simulink model "Pump_comparison"  (R2018b)
settings: Solver=VariableStepAuto  StartTime=0.0  StopTime=200  MaxStep=5  RelTol=1e-3  EnableMultiTasking=on
undefined symbols (not defined in the file): ID, MassFlow, path_carnot, Pressure, Temperature, Water
libraries: carnot x8, simulink x1
settings Model: Creator=drhf  LastModifiedBy=drhf
settings DataIOCC: LimitDataPoints=on  SaveFormat=Array  SignalLoggingSaveFormat=ModelDataLogs
settings OptimizationCC: ExpressionDepthLimit=2147483647  LifeSpan=inf
settings DebuggingCC: UnderspecifiedInitializationDetection=Classic  MergeDetectMultiDrivingBlocksExec=none  SolverPrmCheckMsg=warning  StateNameClashWarn=warning  SFUnexpectedBacktrackingDiag=warning  SFNoUnconditionalDefaultTransitionDiag=warning  SFExecutionAtInitializationDiag=none
settings HardwareCC: ProdBitPerPointer=32  ProdBitPerSizeT=32  ProdBitPerPtrDiffT=32  ProdLargestAtomicFloat=None  ProdIntDivRoundTo=Undefined  ProdEndianess=Unspecified  ProdWordSize=32  ProdHWDeviceType=32-bit Generic
settings ModelReferenceCC: PropagateSignalLabelsOutOfModel=off
settings SFSimCC: SimUseLocalCustomCode=off
settings RTWCC: RTWUseLocalCustomCode=off
settings CodeAppCC: StateflowObjectComments=on
settings GRTTargetCC: TargetLangStandard=C89/C90 (ANSI)  GeneratePreprocessorConditionals=Disable all  CombineOutputUpdateFcns=off  GRTInterface=on
settings ConfigComp: CovMetricSettings=dw  CovHtmlReporting=on  CovSaveCumulativeToWorkspaceVar=on  CovSaveSingleToWorkspaceVar=on  CovExternalEMLEnable=off

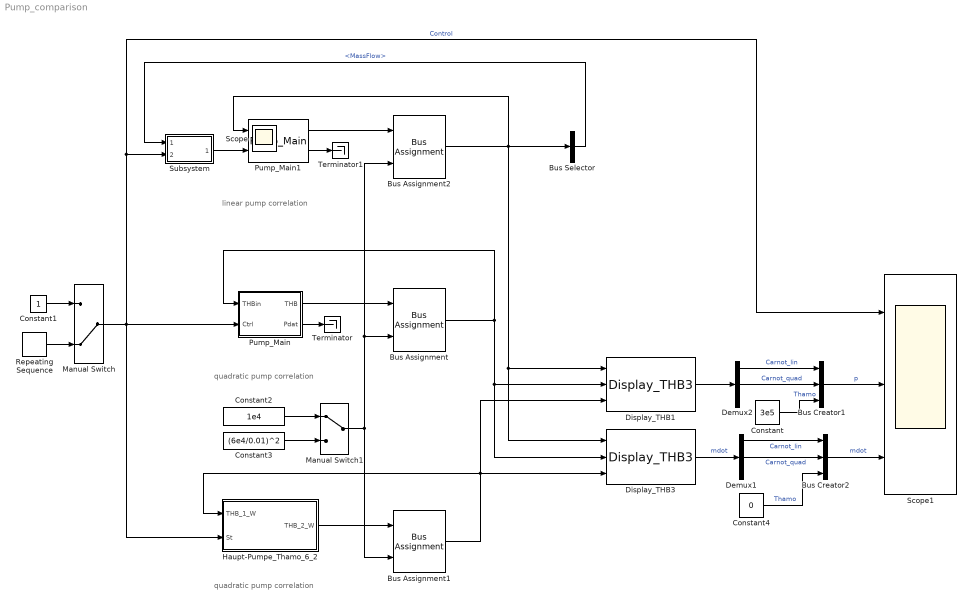
== system Pump_comparison ==
  note: quadratic pump correlation
  note: quadratic pump correlation
  note: linear pump correlation
  Bus Assignment : BusAssignment  AssignedSignals=DPQuadratic
  Bus Assignment1 : BusAssignment  AssignedSignals=DPQuadratic
  Bus Assignment2 : BusAssignment  AssignedSignals=DPQuadratic
  Bus Creator1 : BusCreator  Inputs=3
  Bus Creator2 : BusCreator  Inputs=3
  Bus Selector : BusSelector  OutputSignals=MassFlow
  Constant : Constant  Value=3e5
  Constant1 : Constant
  Constant2 : Constant  Value=1e4
  Constant3 : Constant  Value=(6e4/0.01)^2
  Constant4 : Constant  Value=0
  Demux1 : Demux  Outputs=3
  Demux2 : Demux  Outputs=3
  Display_THB1 : carnot/Outputs/Display_THB3  t=off  m=off  p=on  id=off  mix=off  d=off
      settings: SourceProductName=Carnot
  Display_THB3 : carnot/Outputs/Display_THB3  t=off  m=on  p=off  id=off  mix=off  d=off
      settings: SourceProductName=Carnot
  Haupt-Pumpe_Thamo_6_2 : Subsystem  mask(main pump){a0=60000, a1=43200, a2=0, d=0.05, eta_max=80, a=0, mcp=500, p0=3e5, IDchk=off, fluid_id=Water, mix=0}
      mask prompts: a0 "Konstanter Kennlinienkoeffizient a0 [Pa]"; a1 "Linearer Kennlinienkoeffizient a1 [Pa*s/kg]"; a2 "Quadratischer Kennlinienkoeffizient a2 [Pa*(s/kg)²]"; d "Anschlussdurchmesser [m]"; eta_max "Max. Wirkungsgrad in %"; a "Wirkungsgradexponent"; mcp "Wärmekapazität in J/K"; p0 "Anlagendruck in Pa"; IDchk "Statischen Druck im System berücksichtigen?"; fluid_id "Fluid"; mix "Mischverhältnis Fluid [0..1]"
      mask help:
      | This is the main pump in a circuit. Every circuit must have exactly ONE 'Pump_Main'. Use the 'pump_additional' blocks if you want to use more pumps.
      | Calculate massflow by solving the equations:
      |     pressure_drop = c + l*mdot + q*(mdot)²
      |     pump_pressure = a0 + a1*mdot +a2*(mdot)²
      |     with: pressure_drop = pump_pressure
      | The system pressure specified as parameter is the pressure at the outlet of the pump. All pressure drops in the circuit will reduce this pressure.
      mask init:
      | ID = IDchk*10000+10001;
      mask Help: web(fullfile(path_carnot('help'),'Pump_Main.html'),'-helpbrowser')
      mask TypeOptions fluid_id: Water | Air | Cotton Oil | Silicone Oil | Water-Glycol Mix | Tyfocor LS | Water (Constant 20°C) | Air (dry+ constant 20°C)
      mask DialogControl ParameterTabVar0 Prompt: Hydraulik
      mask DialogControl Container7 Prompt: Thermisch
      mask DialogControl ParameterTabVar01 Prompt: System
      mask Display:
      | plot(-20,0,100,100,[40,70,40,30,30,40,60,70,70,60,40]*0.8,[70,50,30,40,60,70,70,60,40,30,30]*0.8)
      | 
      | port_label('input',1,'THB_1_W')
      | port_label('input',2,'St')
      | port_label('output',1,'THB_2_W')
      | port_label('output',2,'P')
  Manual Switch : ManualSwitch  CurrentSetting=0
  Manual Switch1 : ManualSwitch
  Pump_Main : Subsystem  AncestorBlock=carnot/Hydraulics/Pump_Main  mask(Pump Main){Tini=20, p0=3e5, IDpreset=pressure drop, fluid=Water, mix=0, mix2=0, mix3=0, t1=1, PathName=fullfile(path_carnot('libsl'), 'Hydraulics', 'Pump_Main', 'parameter_set'), FileName='Pump6m.mat', userPath=off, userParam=off, a0=60000, a1=-43200, a2=0, dia=0.025, UA=1, mcp=4182, e0=50, e1=28.8, e2=-10.368}
      mask prompts: Tini "Ambient temperature for losses and initial temperture in °C"; p0 "System pressure at pump inlet [Pa]"; IDpreset "Pressure calculation"; mix "Fluid mixture    [0..1]"; mix2 "Fluid mixture 2 [0..1]"; mix3 "Fluid mixture 3 [0..1]"; t1 "Time constant [s] of PT1 transfer function for massflow"; PathName "Path"; FileName "Parameter set"; userPath "Edit path and name of parameter set"; userParam "User defined parameters"; a0 "a0: pump head in [Pa] (pressure increase at zero flow)"; a1 "a1: pump characteristic linear coefficient [Pa*s/kg]"; a2 "a2: pump characteristic quadratic coefficient [Pa*(s/kg)²]"; dia "Diameter at in- and outlet [m]"; UA "UA: thermal loss coefficient in W/K"; mcp "mcp: thermal capacity of the node in J/K"; e0 "e0: constant coefficient in W"; e1 "e1: linear coefficient in W*s/kg"; e2 "e2: quadratic coefficient in W*(s/kg)²"
      mask help:
      | This is the main pump in a circuit. Every circuit must have exactly ONE 'Pump_Main'. Use the 'Pump_Additional' blocks if you want to use more pumps.
      | The Pump_Main calculate massflow by setting pressure drop in the circuit (dp_circuit) equal to the pressure increase of the pump (pump_head).
      |   dp_circuit = c + l*mdot + q*mdot²
      |   pump_head_ = a0*Ctrl² + a1*Ctrl*mdot +a2*mdot²
      | with
      |   mdot : massflow in kg/s
      |   Ctrl : Control signal input [0..1]
      mask init:
      | % callback to set parameters of model
      | [ok, param] = CarnotCallbacks_PumpMain('SetParameters',gcbh,PathName,FileName);
      mask Help: web(fullfile(path_carnot('help'),'Pump_Main.html'),'-helpbrowser')
      mask TypeOptions Tini: ThermalNodeTHB/Tini
      mask TypeOptions p0: basic_THB/p
      mask TypeOptions IDpreset: ID/IDpreset
      mask TypeOptions fluid: basic_THB/fluid
      mask TypeOptions mix: basic_THB/mix
      mask TypeOptions mix2: basic_THB/mix2
      mask TypeOptions mix3: basic_THB/mix3
      mask TypeOptions t1: Transfer Fcn/t1
      mask Callback userPath: [ok, param] = CarnotCallbacks_PumpMain('UserEdit',gcbh);
      mask Callback userParam: [ok, param] = CarnotCallbacks_PumpMain('UserEdit',gcbh);
      mask TypeOptions a0: PumpHead/Gain
      mask TypeOptions a1: PumpLinear/Value
      mask TypeOptions a2: PumpQuadratic/Value
      mask TypeOptions dia: basic_THB/dia
      mask TypeOptions UA: ThermalNodeTHB/UA
      mask TypeOptions mcp: ThermalNodeTHB/mcp
      mask TypeOptions e0: ElectricConsumptionPump/e0
      mask TypeOptions e1: ElectricConsumptionPump/e1
      mask TypeOptions e2: ElectricConsumptionPump/e2
      mask DialogControl ParameterGroupFile Prompt: Picking a parameter set
      mask DialogControl Control1 Prompt: Carnot public data
      mask DialogControl Control1 Callback: [ok, file] = CarnotCallbacks_PumpMain('GetFilename',gcbh,'public');
      mask DialogControl Control3 Prompt: Carnot internal data
      mask DialogControl Control3 Callback: [ok, file] = CarnotCallbacks_PumpMain('GetFilename',gcbh,'internal');
      mask DialogControl Control4 Prompt: Selected path
      mask DialogControl Control4 Callback: [ok, file] = CarnotCallbacks_PumpMain('GetFilename',gcbh,'selected');
      mask DialogControl PrameterGroupUser Prompt: Parameter Values
      mask DialogControl Container9 Prompt: Hydraulic
      mask DialogControl Container7 Prompt: Thermal
      mask DialogControl Control9 Prompt: Thermal node for temperature:  mcp * dTnode/dt = UA*(Tamb-Tnode) + mdot*cp_in*(Tin-Tnode)
      mask DialogControl Container14 Prompt: Electric
      mask DialogControl Control7 Prompt: Power consumption  Pel = e0 + e1*mdot + e2*mdot²
      mask DialogControl Control5 Prompt: Save in Carnot internal data
      mask DialogControl Control5 Callback: [ok, param] = CarnotCallbacks_PumpMain('SaveFilename',gcbh,'internal','B');
      mask DialogControl Control6 Prompt: Save in selected path
      mask DialogControl Control6 Callback: [ok, param] = CarnotCallbacks_PumpMain('SaveFilename',gcbh,'selected','B');
      mask Display:
      | % user defined picture file
      | picfile = fullfile(path_carnot('intlibsl'), ...
      |         'Hydraulics', 'Pump_Main', 'PumpMain.jpg');
      | 
      | pic = false;
      | if ~BlockIsInCarnotLibrary    % if not located in library any more
      |     if exist(picfile,'file') % show internal picture if defined
      |         image(imread(picfile), [0.2, 0, 0.6, 1])
      |         set_param(gcb, 'BackgroundColor', 'White')
      |         pic = true;
      |     end
      | end
      | if ~pic    % show public picture
      |     set_param(gcb, 'BackgroundColor', 'green')
      |     plot(0,0,1,1,[40,70,40,30,30,40,60,70,70,60,40]/100, ...
      |         [70,50,30,40,60,70,70,60,40,30,30]/100)
      |     disp('main')
      | end
  Pump_Main1 : carnot/Hydraulics/Pump_Main  Tini=20  p0=3e5  IDpreset=pressure drop  fluid=Water  mix=0  mix2=0  mix3=0  t1=1  PathName=fullfile(path_carnot('libsl'), 'Hydraulics', 'Pump_Main', 'parameter_set')  FileName='Pump6m.mat'  userPath=off  userParam=off  a0=60000  a1=-43200  a2=0  dia=0.025  UA=1  mcp=4182  e0=50  e1=28.8  e2=-10.368
      settings: SourceProductName=Carnot
  Repeating Sequence : simulink/Sources/Repeating Sequence  rep_seq_t=[0 20 60 120 180 200]  rep_seq_y=[0 0 1 1 0 0]
  Scope1 : Scope  NumInputPorts=3
  Subsystem : Subsystem
  Terminator : Terminator
  Terminator1 : Terminator
  Scope : Scope
  wires:
  Manual Switch/1 -> Scope1/1, Subsystem/2(Control), Haupt-Pumpe_Thamo_6_2/2(St), Pump_Main/2(Ctrl)  "Control"
  Pump_Main/2(Pdat) -> Terminator/1
  Bus Assignment/1 -> Pump_Main/1(THBin), Display_THB1/2, Display_THB3/2
  Display_THB1/1 -> Demux2/1
  Bus Creator1/1 -> Scope1/2  "p"
  Repeating Sequence/1 -> Manual Switch/2
  Constant1/1 -> Manual Switch/1
  Bus Assignment1/1 -> Display_THB3/3, Haupt-Pumpe_Thamo_6_2/1(THB_1_W), Display_THB1/3
  Manual Switch1/1 -> Bus Assignment2/2, Bus Assignment/2, Bus Assignment1/2
  Bus Creator2/1 -> Scope1/3  "mdot"
  Pump_Main/1(THB) -> Bus Assignment/1
  Haupt-Pumpe_Thamo_6_2/1(THB_2_W) -> Bus Assignment1/1
  Constant2/1 -> Manual Switch1/1
  Constant3/1 -> Manual Switch1/2
  Demux1/1 -> Bus Creator2/1  "Carnot_lin"
  Demux1/2 -> Bus Creator2/2  "Carnot_quad"
  Display_THB3/1 -> Demux1/1  "mdot"
  Pump_Main1/1 -> Bus Assignment2/1
  Pump_Main1/2 -> Terminator1/1
  Bus Assignment2/1 -> Pump_Main1/1, Bus Selector/1, Display_THB3/1, Display_THB1/1
  Constant4/1 -> Bus Creator2/3  "Thamo"
  Constant/1 -> Bus Creator1/3  "Thamo"
  Demux2/2 -> Bus Creator1/2  "Carnot_quad"
  Demux2/1 -> Bus Creator1/1  "Carnot_lin"
  Subsystem/1(Out1) -> Pump_Main1/2
  Bus Selector/1 -> Subsystem/1(mdot)  "<MassFlow>"

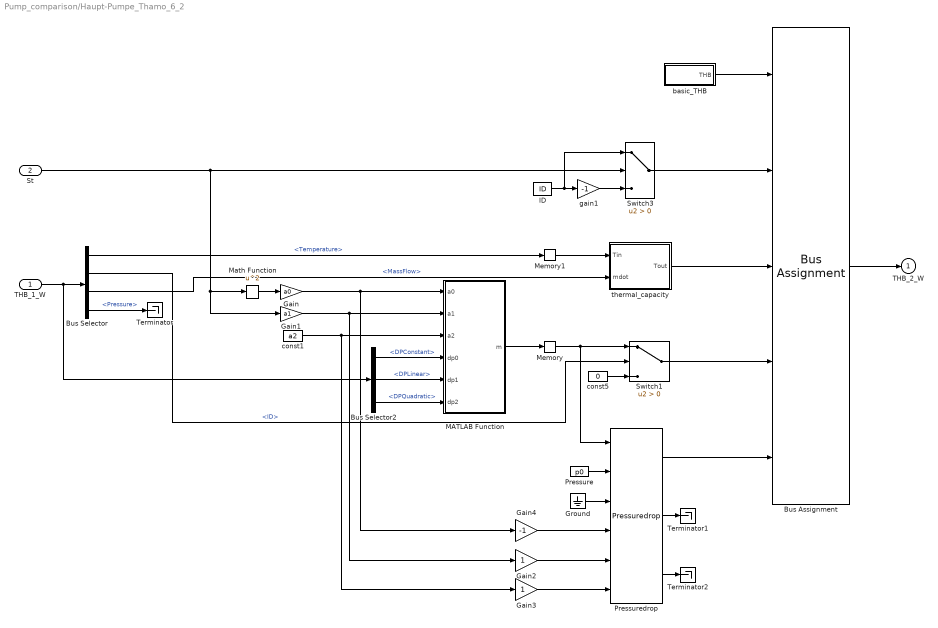
== system Pump_comparison/Haupt-Pumpe_Thamo_6_2 ==
  THB_1_W : Inport
  St : Inport  Port=2
  Bus Assignment : BusAssignment  AssignedSignals=ID,Temperature,MassFlow,Pressure
  Bus Selector : BusSelector  OutputSignals=Temperature,ID,MassFlow,Pressure
  Bus Selector2 : BusSelector  OutputSignals=DPConstant,DPLinear,DPQuadratic
  Gain : Gain  Gain=a0
  Gain1 : Gain  Gain=a1
  Gain2 : Gain
  Gain3 : Gain
  Gain4 : Gain  Gain=-1
  Ground : Ground
  ID : Constant  Value=ID
  MATLAB Function : MATLAB Function  TreatAsAtomicUnit=on
  Math Function : Math  Operator=square  SaturateOnIntegerOverflow=on
  Memory : Memory  InitialCondition=10^-9
  Memory1 : Memory  InitialCondition=20
  Pressure : Constant  Value=p0
  Pressuredrop : carnot/Basic/Pressure_Drop/Pressuredrop
      settings: SourceProductName=Carnot
  Switch1 : Switch  Criteria=u2 > Threshold  SaturateOnIntegerOverflow=on  InputSameDT=on
  Switch3 : Switch  Criteria=u2 > Threshold  SaturateOnIntegerOverflow=on  InputSameDT=on
  Terminator : Terminator
  Terminator1 : Terminator
  Terminator2 : Terminator
  basic_THB : Subsystem  mask(basic THB){t=20, mdot=0, p=p0, ID=Pressure Drop from Massflow, fluid=Water, mix=mix, mix2=0, mix3=0, dia=d, hgt=0}
      mask prompts: t "temperature [°C]"; mdot "massflow [kg/s]"; p "pressure [Pa]"; ID "ID for pressure drop calculation"; mix "fluid mixture [0..1]"; mix2 "fluid mixture 2 [0..1]"; mix3 "fluid mixture 3 [0..1]"; dia "diameter [m]"; hgt "Static height in m"
      mask help:
      | Create a constant Thermo-Hydraulic-Vector.
      | Pressure drop calculation mode (defined by ID):
      |     1 ..  9999 no pressure drop (dp)
      | 10001 .. 19999 dp caused by flowrate
      | 20001 .. inf   dp by flowrate and static height
      mask Help: web(fullfile(path_carnot('help'),'basic_THB.html'),'-helpbrowser')
      mask TypeOptions t: const24/Value
      mask TypeOptions mdot: const25/Value
      mask TypeOptions p: const26/Value
      mask TypeOptions ID: const21/mID
      mask TypeOptions fluid: const27/fluid
      mask TypeOptions mix: const28/Value
      mask TypeOptions mix2: const2/Value
      mask TypeOptions mix3: const3/Value
      mask TypeOptions dia: const29/Value
      mask TypeOptions hgt: const1/Value
      mask DialogControl ParameterTabVar0 Prompt: Hydraulic
      mask DialogControl ParameterTabVar01 Prompt: Fluid
      mask DialogControl ParameterTabVar012 Prompt: Geometry
  const1 : Constant  Value=a2
  const5 : Constant  Value=0
  gain1 : Gain  Gain=-1  SaturateOnIntegerOverflow=on  OutDataTypeStr=Inherit: Same as input  ParamDataTypeStr=Inherit: Same as input
  thermal_capacity : Subsystem  mask(Thermal Capacity){}
      mask help: Basic one node model of a thermal mass using the differential equation:
      mask Help: web(fullfile(path_carnot('help'),'Thermal_Capacity.html'),'-helpbrowser')
  THB_2_W : Outport
  wires:
  Memory1/1 -> thermal_capacity/1(Tin)
  Bus Selector2/3 -> MATLAB Function/6(dp2)  "<DPQuadratic>"
  Bus Selector2/2 -> MATLAB Function/5(dp1)  "<DPLinear>"
  Bus Selector2/1 -> MATLAB Function/4(dp0)  "<DPConstant>"
  MATLAB Function/1(m) -> Memory/1
  Memory/1 -> Pressuredrop/1, Switch1/1
  Gain1/1 -> Gain2/1, MATLAB Function/2(a1)
  Math Function/1 -> Gain/1
  Bus Selector/3 -> thermal_capacity/2(mdot)  "<MassFlow>"
  THB_1_W/1 -> Bus Selector2/1, Bus Selector/1
  Switch1/1 -> Bus Assignment/4
  Switch3/1 -> Bus Assignment/2
  Bus Assignment/1 -> THB_2_W/1
  basic_THB/1(THB) -> Bus Assignment/1
  const5/1 -> Switch1/3
  gain1/1 -> Switch3/3
  ID/1 -> gain1/1, Switch3/1
  St/1 -> Gain1/1, Math Function/1, Switch3/2
  Bus Selector/2 -> Switch1/2  "<ID>"
  thermal_capacity/1(Tout) -> Bus Assignment/3
  Bus Selector/1 -> Memory1/1  "<Temperature>"
  Bus Selector/4 -> Terminator/1  "<Pressure>"
  Gain2/1 -> Pressuredrop/5
  Gain4/1 -> Pressuredrop/4
  Gain3/1 -> Pressuredrop/6
  Pressure/1 -> Pressuredrop/2
  Ground/1 -> Pressuredrop/3
  Gain/1 -> Gain4/1, MATLAB Function/1(a0)
  Pressuredrop/1 -> Bus Assignment/5
  Pressuredrop/2 -> Terminator1/1
  Pressuredrop/3 -> Terminator2/1
  const1/1 -> MATLAB Function/3(a2), Gain3/1

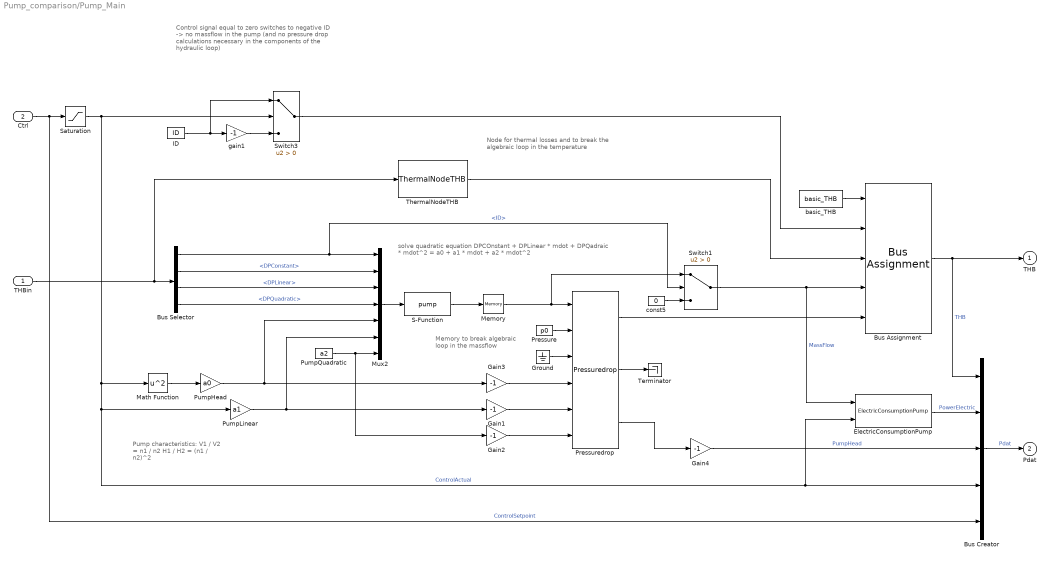
== system Pump_comparison/Pump_Main ==
  note: Node for thermal losses and to break
      | the algebraic loop in the temperature
  note: Memory to
      | break algebraic loop
      | in the massflow
  note: solve quadratic equation
      | DPCOnstant + DPLinear * mdot + DPQadraic * mdot^2
      | = a0 + a1 * mdot + a2 * mdot^2
  note: Control signal equal to zero switches
      | to negative ID -> no massflow in the
      | pump (and no pressure drop calculations
      | necessary in the components of the
      | hydraulic loop)
  note: Pump characteristics:
      | V1 / V2 = n1 / n2
      | H1 / H2 = (n1 / n2)^2
  THBin : Inport
  Ctrl : Inport  Port=2
  Bus Assignment : BusAssignment  AssignedSignals=ID,Temperature,MassFlow,Pressure
  Bus Creator : BusCreator  Inputs=5
  Bus Selector : BusSelector  OutputSignals=ID,DPConstant,DPLinear,DPQuadratic
  ElectricConsumptionPump : carnot/Basic/Hydraulics/ElectricConsumptionPump  e0=e0  e1=e1  e2=e2
      settings: SourceProductName=Carnot
  Gain{1..4} (4 alike) : Gain  Gain=-1
  Ground : Ground
  ID : Constant  Value=ID  mask{IDpreset=pressure drop}
      mask prompts: IDpreset "Calculation"
      mask init:
      | ID = IDpreset*10000 + 1;
      mask TypeOptions IDpreset: pressure drop | pressure drop and pressure head
  Math Function : Math  Operator=square  SaturateOnIntegerOverflow=on
  Memory : Memory
  Mux2 : Mux  Inputs=7
  Pressure : Constant  Value=p0
  Pressuredrop : carnot/Basic/Pressure_Drop/Pressuredrop
      settings: SourceProductName=Carnot
  PumpHead : Gain  Gain=a0
  PumpLinear : Gain  Gain=a1
  PumpQuadratic : Constant  Value=a2
  S-Function : S-Function  FunctionName=pump  SFunctionDeploymentMode=off  EnableBusSupport=off
  Saturation : Saturate  UpperLimit=1  LowerLimit=0
  Switch1 : Switch  Criteria=u2 > Threshold  SaturateOnIntegerOverflow=on  InputSameDT=on
  Switch3 : Switch  Criteria=u2 > Threshold  SaturateOnIntegerOverflow=on  InputSameDT=on
  Terminator : Terminator
  ThermalNodeTHB : carnot/Basic/Thermal_Models/ThermalNodeTHB  UA=UA  mcp=mcp  Tini=Tini
      settings: SourceProductName=Carnot
  basic_THB : carnot/Basic/Hydraulics/basic_THB  t=20  mdot=0  p=p0  ID=No Pressure Drop  fluid=Water  mix=mix  mix2=mix2  mix3=mix3  dia=dia  hgt=0
      settings: SourceProductName=Carnot
  const5 : Constant  Value=0
  gain1 : Gain  Gain=-1  SaturateOnIntegerOverflow=on  OutDataTypeStr=Inherit: Same as input  ParamDataTypeStr=Inherit: Same as input
  THB : Outport
  Pdat : Outport  Port=2
  wires:
  ElectricConsumptionPump/1 -> Bus Creator/2  "PowerElectric"
  Bus Creator/1 -> Pdat/1  "Pdat"
  THBin/1 -> Bus Selector/1, ThermalNodeTHB/1
  Pressuredrop/3 -> Gain4/1
  Bus Selector/1 -> Switch1/2, Mux2/1  "<ID>"
  Switch1/1 -> Bus Assignment/4, ElectricConsumptionPump/1  "MassFlow"
  Mux2/1 -> S-Function/1
  S-Function/1 -> Memory/1
  PumpLinear/1 -> Gain1/1, Mux2/6
  PumpQuadratic/1 -> Mux2/7, Gain2/1
  PumpHead/1 -> Mux2/5, Gain3/1
  Ctrl/1 -> Saturation/1, Bus Creator/5  "ControlSetpoint"
  ID/1 -> Switch3/1, gain1/1
  gain1/1 -> Switch3/3
  Memory/1 -> Pressuredrop/1, Switch1/1
  const5/1 -> Switch1/3
  basic_THB/1 -> Bus Assignment/1
  Bus Assignment/1 -> THB/1, Bus Creator/1  "THB"
  Switch3/1 -> Bus Assignment/2
  ThermalNodeTHB/1 -> Bus Assignment/3
  Bus Selector/2 -> Mux2/2  "<DPConstant>"
  Bus Selector/3 -> Mux2/3  "<DPLinear>"
  Bus Selector/4 -> Mux2/4  "<DPQuadratic>"
  Pressure/1 -> Pressuredrop/2
  Pressuredrop/1 -> Bus Assignment/5
  Ground/1 -> Pressuredrop/3
  Pressuredrop/2 -> Terminator/1
  Saturation/1 -> Switch3/2, Math Function/1, PumpLinear/1, ElectricConsumptionPump/2, Bus Creator/4  "ControlActual"
  Gain3/1 -> Pressuredrop/4
  Gain1/1 -> Pressuredrop/5
  Gain2/1 -> Pressuredrop/6
  Gain4/1 -> Bus Creator/3  "PumpHead"
  Math Function/1 -> PumpHead/1

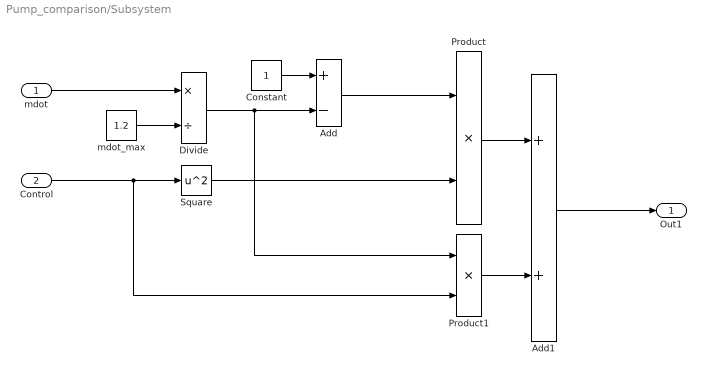
== system Pump_comparison/Subsystem ==
  mdot : Inport
  Control : Inport  Port=2
  Add : Sum  Inputs=+-
  Add1 : Sum
  Constant : Constant
  Divide : Product  Inputs=*/
  Product : Product
  Product1 : Product
  Square : Math  Operator=square  SaturateOnIntegerOverflow=on
  mdot_max : Constant  Value=1.2
  Out1 : Outport
  wires:
  Control/1 -> Product1/2, Square/1
  mdot/1 -> Divide/1
  mdot_max/1 -> Divide/2
  Divide/1 -> Product1/1, Add/2
  Constant/1 -> Add/1
  Add/1 -> Product/1
  Square/1 -> Product/2
  Product/1 -> Add1/1
  Product1/1 -> Add1/2
  Add1/1 -> Out1/1

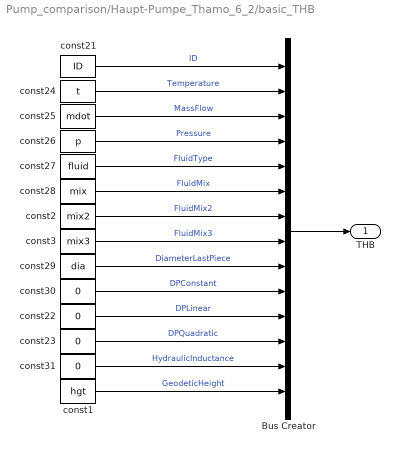
== system Pump_comparison/Haupt-Pumpe_Thamo_6_2/basic_THB ==
  Bus Creator : BusCreator  InitFcn=load THB.mat  Inputs=14  OutDataTypeStr=Bus: THB
  const1 : Constant  Value=hgt
  const2 : Constant  Value=mix2
  const21 : Constant  Value=ID  mask{mID=Pressure Drop from Massflow}
      mask prompts: mID "ID for pressure drop calculation"
      mask init:
      | ID = (mID-1)*10000+1;
      mask TypeOptions mID: No Pressure Drop | Pressure Drop from Massflow | Full Pressure Drop with Static Height
  const{22..23,30..31} (4 alike) : Constant  Value=0
  const24 : Constant  Value=t
  const25 : Constant  Value=mdot
  const26 : Constant  Value=p
  const27 : Constant  Value=fluid  mask{fluid=Water}
      mask TypeOptions fluid: Water | Air | Cotton Oil | Silicone Oil | Water-Glycol Mix | Tyfocor LS | Water (Constant 20°C) | Air (dry+ constant 20°C)
  const28 : Constant  Value=mix
  const29 : Constant  Value=dia
  const3 : Constant  Value=mix3
  THB : Outport
  wires:
  const3/1 -> Bus Creator/8  "FluidMix3"
  const2/1 -> Bus Creator/7  "FluidMix2"
  const1/1 -> Bus Creator/14  "GeodeticHeight"
  const31/1 -> Bus Creator/13  "HydraulicInductance"
  const23/1 -> Bus Creator/12  "DPQuadratic"
  const22/1 -> Bus Creator/11  "DPLinear"
  const29/1 -> Bus Creator/9  "DiameterLastPiece"
  const30/1 -> Bus Creator/10  "DPConstant"
  Bus Creator/1 -> THB/1
  const21/1 -> Bus Creator/1  "ID"
  const24/1 -> Bus Creator/2  "Temperature"
  const25/1 -> Bus Creator/3  "MassFlow"
  const26/1 -> Bus Creator/4  "Pressure"
  const27/1 -> Bus Creator/5  "FluidType"
  const28/1 -> Bus Creator/6  "FluidMix"

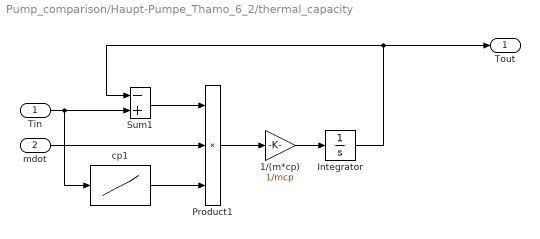
== system Pump_comparison/Haupt-Pumpe_Thamo_6_2/thermal_capacity ==
  Tin : Inport
  mdot : Inport  Port=2
  1/(m*cp) : Gain  Gain=1/mcp  SaturateOnIntegerOverflow=on  OutDataTypeStr=Inherit: Same as input  ParamDataTypeStr=Inherit: Same as input
  Integrator : Integrator  InitialCondition=20
  Product1 : Product  Inputs=3  SaturateOnIntegerOverflow=on  InputSameDT=on  OutDataTypeStr=Inherit: Same as first input
  Sum1 : Sum  Inputs=-+  SaturateOnIntegerOverflow=on  InputSameDT=on  OutDataTypeStr=Inherit: Same as first input
  cp1 : Lookup_n-D  NumberOfTableDimensions=1  BreakpointsForDimension1=[0,10,20,30,40,50,60,70,80,90,100]  Table=[4218,4192,4182,4179,4179,4181,4184,4190,4196,4205,4216]  InternalRulePriority=Speed  RndMeth=Simplest  InputSameDT=on
  Tout : Outport
  wires:
  mdot/1 -> Product1/2
  Tin/1 -> cp1/1, Sum1/2
  Integrator/1 -> Sum1/1, Tout/1
  Product1/1 -> 1/(m*cp)/1
  1/(m*cp)/1 -> Integrator/1
  Sum1/1 -> Product1/1
  cp1/1 -> Product1/3

== matlab function Pump_comparison/Haupt-Pumpe_Thamo_6_2/MATLAB Function ==
  data: a0 input; a1 input; a2 input; m output; dp0 input; dp1 input; dp2 input
function m = fcn(a0,a1,a2,dp0,dp1,dp2)
m =  real(max(roots([a2-dp2 a1-dp1 a0-dp0])));
% v = real(roots([a2-dp2 a1-dp1 a0-dp0]));
% if isempty(v)
%     v = 0;
% end
% m =  max(v);
end
